simulink model "ysw3_32"  (R2014a)
settings: Solver=ode45  StartTime=0.0  StopTime=10.0  RelTol=1e-3
settings Model: Creator=Administrator  LastModifiedBy=Administrator

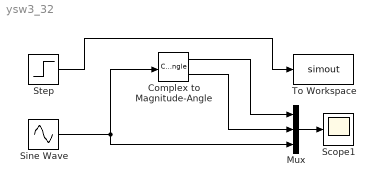
== system ysw3_32 ==
  Complex to Magnitude-Angle : ComplexToMagnitudeAngle
  Mux : Mux  Inputs=3
  Scope1 : Scope
      settings: TimeRange=10
  Sine Wave : Sin  SampleTime=0.1
  Step : Step  SampleTime=0
  To Workspace : ToWorkspace  VariableName=simout  SaveFormat=Timeseries  SampleTime=-1
  wires:
  Mux/1 -> Scope1/1
  Sine Wave/1 -> Mux/3, Complex to Magnitude-Angle/1
  Complex to Magnitude-Angle/1 -> Mux/1
  Complex to Magnitude-Angle/2 -> Mux/2
  Step/1 -> To Workspace/1
